simulink model "testingModeloPromediado"  (R2021a)
settings: Solver=VariableStepAuto  StartTime=0.0  StopTime=10.0  RelTol=1e-3
undefined symbols (not defined in the file or in its folder): CBUS, comp_h2_fc, comp_h2o_fc, comp_o2_fc, I_end_fc, I_nom_fc, Ion, L1, Lithium, p_air_nom_fc, p_fuel_nom_fc, V_0_fc, V_1_fc, V_end_fc, V_nom_fc
libraries: spsSeriesRLCBranchLib x2, spsControlledCurrentSourceLib x2, spsBatteryLib x1, spsControlledVoltageSourceLib x1, spsDiodeLib x1, spsFuelCellStackLib x1, pid_lib x1
settings Model: Creator=leonardopalacios  LastModifiedBy=leonardopalacios

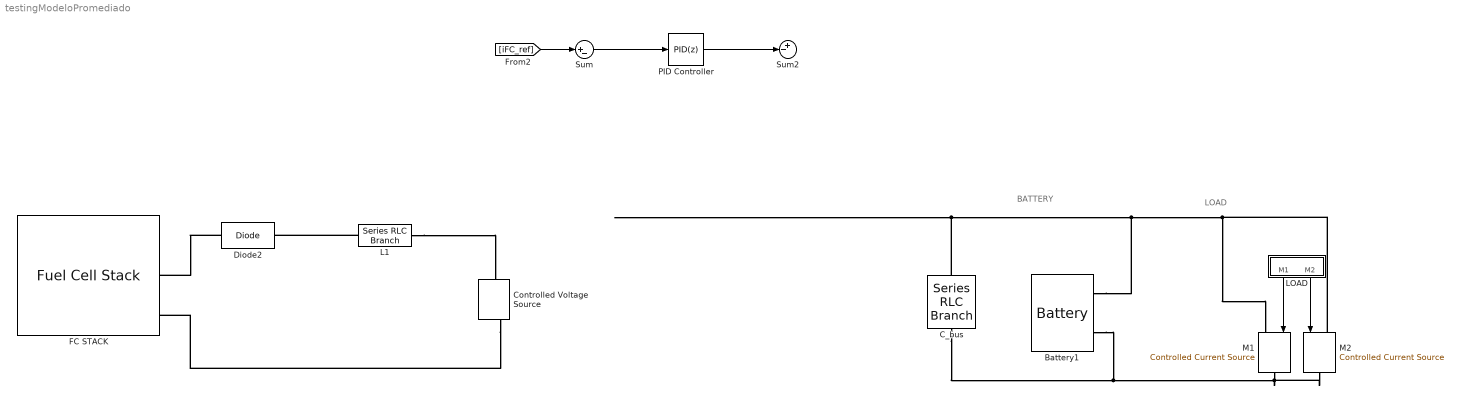
== system testingModeloPromediado ==
  note: BATTERY
  note: LOAD
  Battery1 : spsBatteryLib/Battery  BatType=Lithium-Ion  ShowTempParam=off  ThermalPreset=no  ShowAgeParam=off  NomV=40  NomQ=2.2  SOC=50  Batt_Tr=30  PresetModel=on  MaxQ=2.2  MinV=30  FullV=46.5595  Dis_rate=0.95652  R=0.18182  Normal_OP=1.9896  expZone="[43.2154     0.108087]"  current=[6.5 13 32.5]  Units=Time  Tci=20  NomT=25  T2=0  MaxQ2=2.208  FullV2=3.45  Normal_OP2=2.8  expZone2="[3.22        0.23]"  Rca=0.6  ti=1000  Dp=0  Neq0=0  Tsim=1e6  Ta1=25  Qeol=5.4*0.9  Reol=0.013333*1.2  Char_age=[2.3478, 3]  Dis_age=[2.3478, 10]  N1=1500  N2=10500  N3=1000  N4=1400  Ta2=45  N5=950
  C_bus : spsSeriesRLCBranchLib/Series RLC Branch  LConnTagsString=__new0  RConnTagsString=__new0  BranchType=C  Resistance=1e5  Inductance=1e-3  SetiL0=off  InitialCurrent=0  Capacitance=CBUS  Setx0=on  InitialVoltage=48  Measurements=None
  Controlled Voltage Source : spsControlledVoltageSourceLib/Controlled Voltage Source  Initialize=on  Source_Type=AC  Amplitude=0  Phase=0  Frequency=0  Measurements=None
  Diode2 : spsDiodeLib/Diode  Ron=0.001  Lon=0  Vf=0.8  IC=0  UseSnubber=off  Rs=500  Cs=250e-9  Measurements=off
  FC STACK : spsFuelCellStackLib/Fuel Cell Stack  PresetModel=No (User-Defined)  FcType=0  Detailed=Detailed  Eoc=[V_0_fc V_1_fc]  NomVI=[I_nom_fc V_nom_fc]  EndVI=[I_end_fc V_end_fc]  Nc=cells_fc  n=SE_nom_fc  TOp=T_opt_fc  AirFr=q_air_fc  SuppPress=[p_fuel_nom_fc p_air_nom_fc]  Comp=[comp_h2_fc comp_o2_fc comp_h2o_fc]  SignX=off  SignY=off  FlowRateH2=off  FlowRateAir=off  SystemTemp=off  SystemPH2=off  SystemPAir=off  FCDyn=off  FC_tau=1  Peak_O2=80  V_Under=10
      settings: SourceProductBaseCode=PS
  L1 : spsSeriesRLCBranchLib/Series RLC Branch  LConnTagsString=__new0  RConnTagsString=__new0  BranchType=L  Resistance=1e5  Inductance=L1  SetiL0=off  InitialCurrent=0  Capacitance=1e-6  Setx0=off  InitialVoltage=0  Measurements=None
  LOAD : Subsystem
  M1 : spsControlledCurrentSourceLib/Controlled Current Source  Initialize=off  Source_Type=AC  Amplitude=0  Phase=0  Frequency=0  Measurements=None
  M2 : spsControlledCurrentSourceLib/Controlled Current Source  Initialize=off  Source_Type=AC  Amplitude=0  Phase=0  Frequency=0  Measurements=None
  PID Controller : pid_lib/PID Controller  Controller=PID  Form=Parallel  TimeDomain=Discrete-time  UseExternalTs=off  SampleTime=-1  IntegratorMethod=Forward Euler  FilterMethod=Forward Euler  ControllerParametersSource=internal  P=1  I=10  D=0  UseFilter=on  N=100  TunerSelectOption=Transfer Function Based (PID Tuner App)  InitialConditionSource=internal  InitialConditionForIntegrator=0  InitialConditionForFilter=0  DifferentiatorICPrevScaledInput=0  ExternalReset=none  TrackingMode=off  Kt=1  LimitOutput=off  SatLimitsSource=internal  UpperSaturationLimit=inf  LowerSaturationLimit=-inf  LinearizeAsGain=on  AntiWindupMode=none  Kb=1  POutMin=[]  POutMax=[]  IOutMin=[]  IOutMax=[]  DOutMin=[]  DOutMax=[]  NOutMin=[]  NOutMax=[]  SumOutMin=[]  SumOutMax=[]  SaturationOutMin=[]  SaturationOutMax=[]  PParamMin=[]  PParamMax=[]  IParamMin=[]  IParamMax=[]  DParamMin=[]  DParamMax=[]  NParamMin=[]  NParamMax=[]  KbParamMin=[]  KbParamMax=[]  KtParamMin=[]  KtParamMax=[]  KbOutMin=[]  KbOutMax=[]  KtOutMin=[]  KtOutMax=[]  IntegratorOutMin=[]  IntegratorOutMax=[]  FilterOutMin=[]  FilterOutMax=[]  SumI1OutMin=[]  SumI1OutMax=[]  SumI2OutMin=[]  SumI2OutMax=[]  SumI3OutMin=[]  SumI3OutMax=[]  SumI4OutMin=[]  SumI4OutMax=[]  SumDOutMin=[]  SumDOutMax=[]  DifferentiatorOutMin=[]  DifferentiatorOutMax=[]  FilterDiffOutCoefMin=[]  FilterDiffOutCoefMax=[]  ReciprocalOutMin=[]  ReciprocalOutMax=[]  SumDenOutMin=[]  SumDenOutMax=[]  SumNumOutMin=[]  SumNumOutMax=[]  DivideOutMin=[]  DivideOutMax=[]  UdiffTsProdOutMin=[]  UdiffTsProdOutMax=[]  NTsProdOutMin=[]  NTsProdOutMax=[]  UintegralTsProdOutMin=[]  UintegralTsProdOutMax=[]  UngainTsProdOutMin=[]  UngainTsProdOutMax=[]  IntegratorContinuousStateAttributes=''  IntegratorStateMustResolveToSignalObject=off  IntegratorRTWStateStorageClass=Auto  FilterContinuousStateAttributes=''  FilterStateMustResolveToSignalObject=off  FilterRTWStateStorageClass=Auto  ParallelPVariant=InternalParameters  IdealPVariant=Disabled  IVariant=InternalParameters  DVariant=InternalParameters  IntegratorVariant=Discrete  SatVariant=Disabled  AWVariant=Passthrough  PCopyVariant=Disabled  TRVariant=Disabled  FdbkBlocksVariant=Forward  IdealPFdbkVariant=Disabled  SatFdbkVariant=Disabled  DerivativeFilterVariant=ForwardEulerFilter  NVariant=InternalParameters  NCopyVariant=Disabled  FilterICVariant=InternalICsFilter  IntegratorICVariant=InternalICs  ExternalResetVariant=Disabled  TRSumVariant=Passthrough  SumFdbkVariant=Disabled  SumVariant=Sum_PID  TsampFilterVariant=InternalTs  TsampNgainVariant=Passthrough  TsampIntegralVariant=Passthrough  ExternalSaturationOutDataTypeStr=Inherit: Same as second input
  Sum : Sum  Inputs=|+-
  Sum2 : Sum  Inputs=+-|
  wires:
  LOAD/1(M1) -> M1/1
  LOAD/2(M2) -> M2/1
  [iFC_ref] -> Sum/1
  Sum/1 -> PID Controller/1
  PID Controller/1 -> Sum2/2
  connections:
  Battery1/LConn2 -- C_bus/RConn1 -- M1/RConn1 -- M2/RConn1
  Controlled Voltage Source/LConn1 -- FC STACK/RConn2
  C_bus/LConn1 -- M1/LConn1 -- M2/LConn1 -- Battery1/LConn1
  Diode2/LConn1 -- FC STACK/RConn1
  L1/LConn1 -- Diode2/RConn1
  L1/RConn1 -- Controlled Voltage Source/RConn1

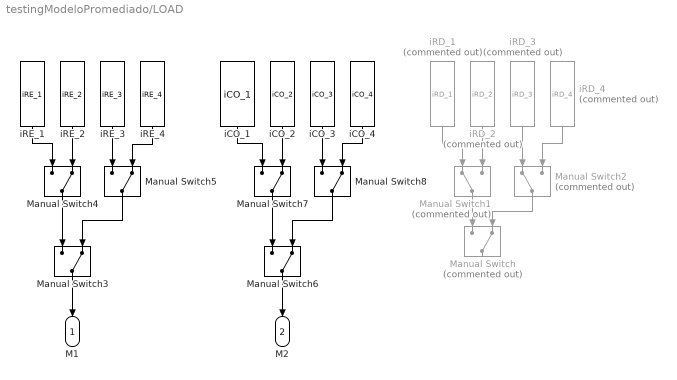
== system testingModeloPromediado/LOAD ==
  Manual Switch : ManualSwitch  Commented=on  CurrentSetting=0
  Manual Switch1 : ManualSwitch  Commented=on
  Manual Switch2 : ManualSwitch  Commented=on
  Manual Switch{3..8} (6 alike) : ManualSwitch  CurrentSetting=0
  iCO_1 : FromWorkspace  VariableName=iCO_1
  iCO_2 : FromWorkspace  VariableName=iCO_2
  iCO_3 : FromWorkspace  VariableName=iCO_3
  iCO_4 : FromWorkspace  VariableName=iCO_4
  iRD_1 : FromWorkspace  Commented=on  VariableName=iRD_1
  iRD_2 : FromWorkspace  Commented=on  VariableName=iRD_2
  iRD_3 : FromWorkspace  Commented=on  VariableName=iRD_3
  iRD_4 : FromWorkspace  Commented=on  VariableName=iRD_4
  iRE_1 : FromWorkspace  VariableName=iRE_1
  iRE_2 : FromWorkspace  VariableName=iRE_2
  iRE_3 : FromWorkspace  VariableName=iRE_3
  iRE_4 : FromWorkspace  VariableName=iRE_4
  M1 : Outport
  M2 : Outport  Port=2
  wires:
  Manual Switch5/1 -> Manual Switch3/2
  iRD_2/1 -> Manual Switch1/2
  iRD_4/1 -> Manual Switch2/2
  iRE_4/1 -> Manual Switch5/2
  Manual Switch4/1 -> Manual Switch3/1
  iCO_1/1 -> Manual Switch7/1
  Manual Switch2/1 -> Manual Switch/2
  iRE_2/1 -> Manual Switch4/2
  iRE_1/1 -> Manual Switch4/1
  iRD_1/1 -> Manual Switch1/1
  Manual Switch8/1 -> Manual Switch6/2
  iCO_3/1 -> Manual Switch8/1
  Manual Switch7/1 -> Manual Switch6/1
  iCO_4/1 -> Manual Switch8/2
  iRE_3/1 -> Manual Switch5/1
  iCO_2/1 -> Manual Switch7/2
  iRD_3/1 -> Manual Switch2/1
  Manual Switch1/1 -> Manual Switch/1
  Manual Switch3/1 -> M1/1
  Manual Switch6/1 -> M2/1
